simulink model "Fuzzy_Control"  (R2023a)
settings: Solver=VariableStepAuto  StartTime=0.0  StopTime=2.5  RelTol=1e-3
libraries: slpidlib x1, fuzblock x1
settings Model: Creator=Νίκος  LastModifiedBy=Νίκος

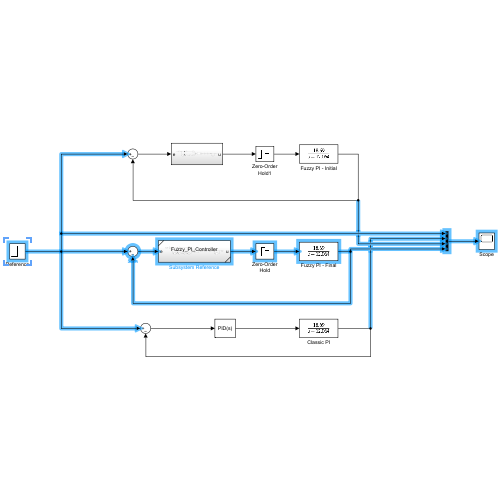
[thumbnail: Simulink's stored preview of the top-level diagram]
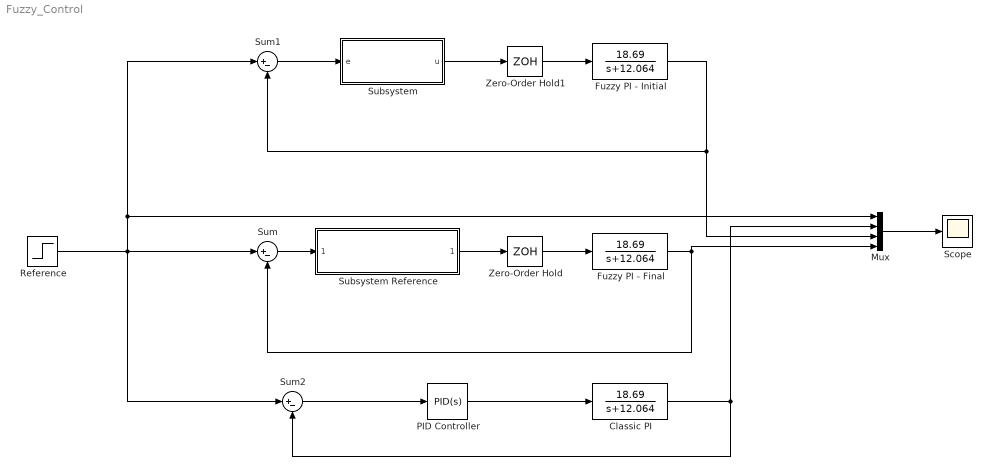
== system Fuzzy_Control ==
  Classic PI : TransferFcn  Numerator=[18.69]  Denominator=[1 12.064]
  Fuzzy PI - Final : TransferFcn  Numerator=[18.69]  Denominator=[1 12.064]
  Fuzzy PI - Initial : TransferFcn  Numerator=[18.69]  Denominator=[1 12.064]
  Mux : Mux
  PID Controller : slpidlib/PID Controller  Controller=PID  Form=Parallel  TimeDomain=Continuous-time  UseExternalTs=off  SampleTime=-1  IntegratorMethod=Forward Euler  FilterMethod=Forward Euler  ControllerParametersSource=internal  P=2  I=12  UseKiTs=off  D=0  N=100  UseFilter=on  TunerSelectOption=Transfer Function Based (PID Tuner App)  InitialConditionSource=internal  InitialConditionForIntegrator=0  InitialConditionForFilter=0  DifferentiatorICPrevScaledInput=0  ExternalReset=none  TrackingMode=off  Kt=1  LimitOutput=off  SatLimitsSource=internal  UpperSaturationLimit=inf  LowerSaturationLimit=-inf  LinearizeAsGain=on  AntiWindupMode=none  Kb=1  LimitIntegrator=off  UpperIntegratorSaturationLimit=inf  LowerIntegratorSaturationLimit=-inf  POutMin=[]  POutMax=[]  IOutMin=[]  IOutMax=[]  DOutMin=[]  DOutMax=[]  NOutMin=[]  NOutMax=[]  SumOutMin=[]  SumOutMax=[]  SaturationOutMin=[]  SaturationOutMax=[]  PParamMin=[]  PParamMax=[]  IParamMin=[]  IParamMax=[]  DParamMin=[]  DParamMax=[]  NParamMin=[]  NParamMax=[]  KbParamMin=[]  KbParamMax=[]  KtParamMin=[]  KtParamMax=[]  KbOutMin=[]  KbOutMax=[]  KtOutMin=[]  KtOutMax=[]  IntegratorOutMin=[]  IntegratorOutMax=[]  FilterOutMin=[]  FilterOutMax=[]  SumI1OutMin=[]  SumI1OutMax=[]  SumI2OutMin=[]  SumI2OutMax=[]  SumI3OutMin=[]  SumI3OutMax=[]  SumI4OutMin=[]  SumI4OutMax=[]  SumDOutMin=[]  SumDOutMax=[]  DifferentiatorOutMin=[]  DifferentiatorOutMax=[]  FilterDiffOutCoefMin=[]  FilterDiffOutCoefMax=[]  ReciprocalOutMin=[]  ReciprocalOutMax=[]  SumDenOutMin=[]  SumDenOutMax=[]  SumNumOutMin=[]  SumNumOutMax=[]  DivideOutMin=[]  DivideOutMax=[]  UdiffTsProdOutMin=[]  UdiffTsProdOutMax=[]  NTsProdOutMin=[]  NTsProdOutMax=[]  UintegralTsProdOutMin=[]  UintegralTsProdOutMax=[]  UngainTsProdOutMin=[]  UngainTsProdOutMax=[]  ClampingZeroOutDataTypeStr=Inherit: Inherit via back propagation  ClampingZeroOutMin=[]  ClampingZeroOutMax=[]  FilterDenConstantOutDataTypeStr=Inherit: Inherit via back propagation  FilterDenConstantOutMin=[]  FilterDenConstantOutMax=[]  PCopyOutDataTypeStr=Inherit: Inherit via back propagation  PCopyOutMin=[]  PCopyOutMax=[]  NCopyOutDataTypeStr=Inherit: Inherit via back propagation  NCopyOutMin=[]  NCopyOutMax=[]  IntegratorContinuousStateAttributes=''  IntegratorStateMustResolveToSignalObject=off  IntegratorRTWStateStorageClass=Auto  FilterContinuousStateAttributes=''  FilterStateMustResolveToSignalObject=off  FilterRTWStateStorageClass=Auto  ParallelPVariant=InternalParameters  IdealPVariant=Disabled  IVariant=InternalParameters  DVariant=InternalParameters  IntegratorVariant=Continuous  SatVariant=Disabled  AWVariant=Passthrough  PCopyVariant=Disabled  TRVariant=Disabled  FdbkBlocksVariant=Forward  IdealPFdbkVariant=Disabled  SatFdbkVariant=Disabled  DerivativeFilterVariant=ContFilter  NVariant=InternalParameters  NCopyVariant=Disabled  FilterICVariant=InternalICsFilter  IntegratorICVariant=InternalICs  ExternalResetVariant=Disabled  TRSumVariant=Passthrough  SumFdbkVariant=Disabled  SumVariant=Sum_PID  TsampFilterVariant=InternalTs  TsampNgainVariant=Passthrough  TsampIntegralVariant=Disabled_SignalSpec  ExternalSaturationOutDataTypeStr=Inherit: Same as second input
  Reference : Step  Time=0  SampleTime=0.01
  Scope : Scope
  Subsystem : Subsystem
  Subsystem Reference : Subsystem  ReferencedSubsystem=Fuzzy_PI_Controller
  Sum : Sum  Inputs=|+-
  Sum1 : Sum  Inputs=|+-
  Sum2 : Sum  Inputs=|+-
  Zero-Order Hold : ZeroOrderHold  SampleTime=-1
  Zero-Order Hold1 : ZeroOrderHold  SampleTime=-1
  wires:
  Zero-Order Hold/1 -> Fuzzy PI - Final/1
  Fuzzy PI - Final/1 -> Mux/4, Sum/2
  Mux/1 -> Scope/1
  Sum/1 -> Subsystem Reference/1
  Subsystem Reference/1 -> Zero-Order Hold/1
  Fuzzy PI - Initial/1 -> Mux/3, Sum1/2
  Reference/1 -> Sum2/1, Sum1/1, Mux/1, Sum/1
  Zero-Order Hold1/1 -> Fuzzy PI - Initial/1
  Classic PI/1 -> Mux/2, Sum2/2
  Sum2/1 -> PID Controller/1
  PID Controller/1 -> Classic PI/1
  Sum1/1 -> Subsystem/1(e)
  Subsystem/1(u) -> Zero-Order Hold1/1

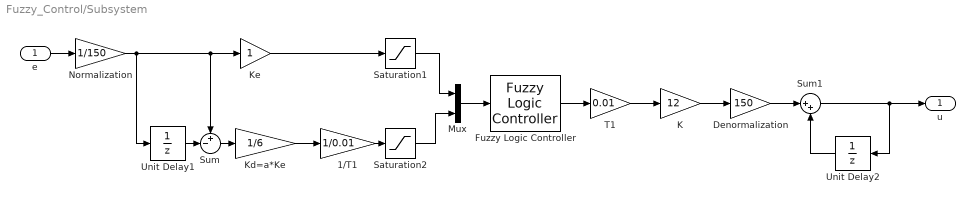
== system Fuzzy_Control/Subsystem ==
  e : Inport
  1/T1 : Gain  Gain=1/0.01
  Denormalization : Gain  Gain=150
  Fuzzy Logic Controller : fuzblock/Fuzzy Logic  Controller  FIS='Fuzzy_Controller.fis'  OutputSampleNumber=101  DataType=double  FuzzifiedInputs=off  RuleFiringStrengths=off  RuleOutputs=off  AggregatedOutputs=off  SimulateUsing=Interpreted execution  OutOfRangeInputValueMessage=warning  NoRuleFiredMessage=warning  EmptyOutputFuzzySetMessage=warning
  K : Gain  Gain=12
  Kd=a*Ke : Gain  Gain=1/6
  Ke : Gain
  Mux : Mux  Inputs=2
  Normalization : Gain  Gain=1/150
  Saturation1 : Saturate
  Saturation2 : Saturate
  Sum : Sum  Inputs=+-|
  Sum1 : Sum  Inputs=|++
  T1 : Gain  Gain=0.01
  Unit Delay1 : UnitDelay  SampleTime=-1  HasFrameUpgradeWarning=on
  Unit Delay2 : UnitDelay  SampleTime=-1  HasFrameUpgradeWarning=on
  u : Outport
  wires:
  Unit Delay2/1 -> Sum1/2
  Sum1/1 -> u/1, Unit Delay2/1
  Fuzzy Logic Controller/1 -> T1/1
  Saturation2/1 -> Mux/2
  K/1 -> Denormalization/1
  Mux/1 -> Fuzzy Logic Controller/1
  Ke/1 -> Saturation1/1
  1/T1/1 -> Saturation2/1
  T1/1 -> K/1
  e/1 -> Normalization/1
  Sum/1 -> Kd=a*Ke/1
  Normalization/1 -> Unit Delay1/1, Sum/1, Ke/1
  Saturation1/1 -> Mux/1
  Kd=a*Ke/1 -> 1/T1/1
  Denormalization/1 -> Sum1/1
  Unit Delay1/1 -> Sum/2
